simulink model "trajectory_plot"  (R2021a)
settings: Solver=FixedStepAuto  StartTime=0.0  StopTime=sim_time  RelTol=1e-3
values from neighbouring files (symbols this model uses):
  mjd2000_dep = MA.SC1.mjd2000_dep    [main_video_sim.m]
  TrajSC = [TrajSC, time_mjd2000_traj']    [main_video_sim.m]
undefined symbols (not defined in the file or in its folder): adim, planet_eph
libraries: vrlib x1
settings Model: SimulationMode=accelerator  Creator=enric  LastModifiedBy=enric

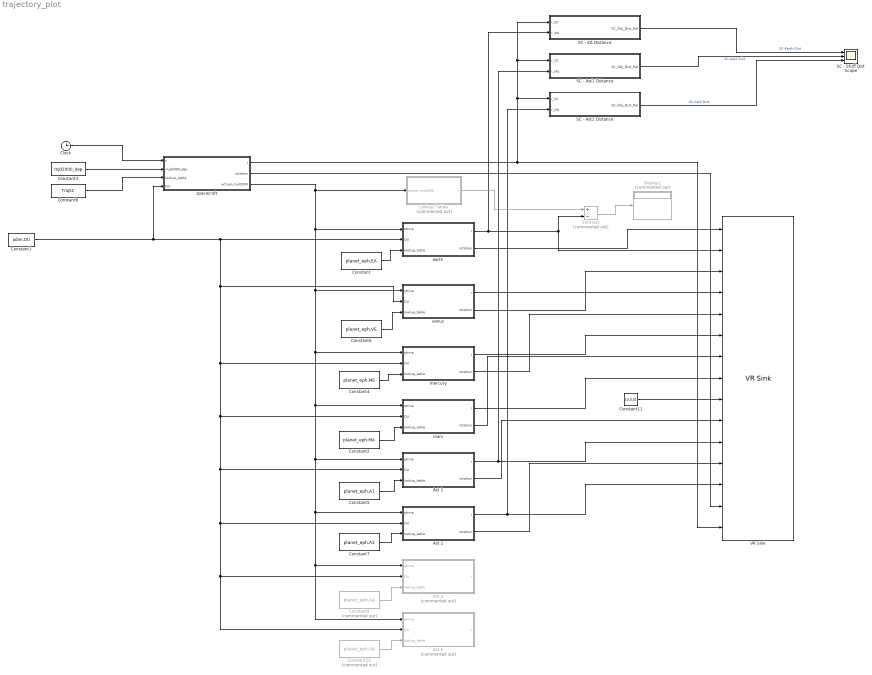
== system trajectory_plot ==
  Ast 1 : MATLAB Function  TreatAsAtomicUnit=on
  Ast 2 : MATLAB Function  TreatAsAtomicUnit=on
  Ast a : MATLAB Function  Commented=on  TreatAsAtomicUnit=on
  Ast b : MATLAB Function  Commented=on  TreatAsAtomicUnit=on
  Clock : Clock
  Constant : Constant  Value=planet_eph.EA
  Constant1 : Constant  Value=adim.DU
  Constant10 : Constant  Commented=on  Value=planet_eph.Ab
  Constant11 : Constant  Value=[0,0,5]
  Constant2 : Constant  Value=planet_eph.MA
  Constant3 : Constant  Value=mjd2000_dep
  Constant4 : Constant  Value=planet_eph.ME
  Constant5 : Constant  Value=planet_eph.A1
  Constant6 : Constant  Value=planet_eph.VE
  Constant7 : Constant  Value=planet_eph.A2
  Constant8 : Constant  Value=TrajSC
  Constant9 : Constant  Commented=on  Value=planet_eph.Aa
  Display1 : Display  Commented=on
  Lookup Tables : Subsystem  Commented=on
  SC - Ast1 Distance : MATLAB Function  TreatAsAtomicUnit=on
  SC - Ast2 Distance : MATLAB Function  TreatAsAtomicUnit=on
  SC - EA Distance : MATLAB Function  TreatAsAtomicUnit=on
  SC - Stuff Dist Scope : Scope  NumInputPorts=3
  Subtract : Sum  Commented=on  Inputs=+-
  VR Sink : vrlib/VR Sink  InstantiateOnLoad=on  SampleTime=0.1  ViewEnable=on  RemoteChange=off  RemoteView=off  FieldsWritten=Earth.rotation.4.1.1.double#Earth.translation.3.1.1.double#Venus.rotation.4.1.1.double#Venus.translation.3.1.1.double#Mercury.rotation.4.1.1.double#Mercury.translation.3.1.1.double#Mars.rotation.4.1.1.double#Mars.translation.3.1.1.double#Luigi.position.3.1.1.double#Golevka.rotation.4.1.1.double#Golevka.translation.3.1.1.double#Tautatis.rotation.4.1.1.double#Tautatis.translation.3.1.1.double#Hayabusa2.rotation.4.1.1.double#Hayabusa2.translation.3.1.1.double  WorldFileName=inner_solar_system.x3d  AutoView=on  VideoDimensions=[]  AllowVariableSize=off
  earth : MATLAB Function  TreatAsAtomicUnit=on
  mars : MATLAB Function  TreatAsAtomicUnit=on
  mercury : MATLAB Function  TreatAsAtomicUnit=on
  spacecraft : MATLAB Function  TreatAsAtomicUnit=on
  venus : MATLAB Function  TreatAsAtomicUnit=on
  wires:
  earth/1(r) -> SC - EA Distance/2(r_obj), VR Sink/2, Subtract/2
  Constant/1 -> earth/3(lookup_table)
  Constant2/1 -> mars/3(lookup_table)
  mars/1(r) -> VR Sink/8
  Constant4/1 -> mercury/3(lookup_table)
  mercury/1(r) -> VR Sink/6
  Constant1/1 -> mars/2(DU), Ast 2/2(DU), Ast b/2(DU), Ast a/2(DU), Ast 1/2(DU), mercury/2(DU), venus/2(DU), earth/2(DU), spacecraft/4(DU)
  Constant6/1 -> venus/3(lookup_table)
  venus/1(r) -> VR Sink/4
  Constant8/1 -> spacecraft/3(lookup_table)
  Clock/1 -> spacecraft/1(t)
  Constant3/1 -> spacecraft/2(mjd2000_dep)
  spacecraft/3(actual_mjd2000) -> earth/1(qtime), mars/1(qtime), Ast 1/1(qtime), Ast 2/1(qtime), Ast b/1(qtime), Ast a/1(qtime), mercury/1(qtime), venus/1(qtime), Lookup Tables/1(actual mjd2000)
  Constant5/1 -> Ast 1/3(lookup_table)
  Constant7/1 -> Ast 2/3(lookup_table)
  Constant9/1 -> Ast a/3(lookup_table)
  Constant10/1 -> Ast b/3(lookup_table)
  Ast 1/1(r) -> VR Sink/11, SC - Ast1 Distance/2(r_obj)
  Ast 2/1(r) -> SC - Ast2 Distance/2(r_obj), VR Sink/13
  spacecraft/1(r) -> VR Sink/15, SC - EA Distance/1(r_SC), SC - Ast1 Distance/1(r_SC), SC - Ast2 Distance/1(r_SC)
  Lookup Tables/1(r) -> Subtract/1
  Subtract/1 -> Display1/1
  earth/2(rotation) -> VR Sink/1
  venus/2(rotation) -> VR Sink/3
  mercury/2(rotation) -> VR Sink/5
  Ast 2/2(rotation) -> VR Sink/12
  Ast 1/2(rotation) -> VR Sink/10
  mars/2(rotation) -> VR Sink/7
  Constant11/1 -> VR Sink/9
  spacecraft/2(rotation) -> VR Sink/14
  SC - EA Distance/1(SC_Obj_Dist_Rel) -> SC - Stuff Dist Scope/1  "SC-Earth Dist"
  SC - Ast1 Distance/1(SC_Obj_Dist_Rel) -> SC - Stuff Dist Scope/2  "SC-Ast1 Dist"
  SC - Ast2 Distance/1(SC_Obj_Dist_Rel) -> SC - Stuff Dist Scope/3  "SC-Ast2 Dist"

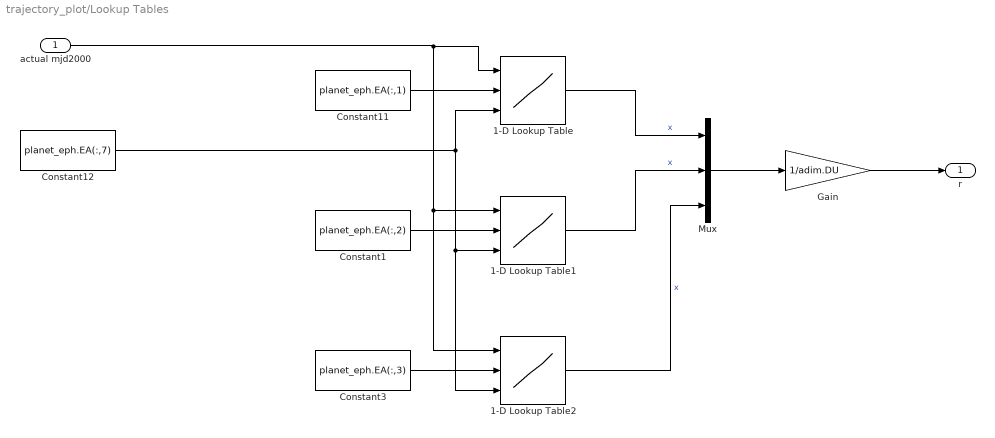
== system trajectory_plot/Lookup Tables ==
  actual mjd2000 : Inport
  1-D Lookup Table : Lookup_n-D  NumberOfTableDimensions=1  BreakpointsForDimension1Source=Input port  BreakpointsForDimension1=[7]  TableSource=Input port  Table=tanh([-5:5])  InternalRulePriority=Speed  RndMeth=Simplest  InputSameDT=on
      settings: InputPortMap=u0,p221,p5
  1-D Lookup Table1 : Lookup_n-D  NumberOfTableDimensions=1  BreakpointsForDimension1Source=Input port  BreakpointsForDimension1=[7]  TableSource=Input port  Table=tanh([-5:5])  InternalRulePriority=Speed  RndMeth=Simplest  InputSameDT=on
      settings: InputPortMap=u0,p221,p5
  1-D Lookup Table2 : Lookup_n-D  NumberOfTableDimensions=1  BreakpointsForDimension1Source=Input port  BreakpointsForDimension1=[7]  TableSource=Input port  Table=tanh([-5:5])  InternalRulePriority=Speed  RndMeth=Simplest  InputSameDT=on
      settings: InputPortMap=u0,p221,p5
  Constant1 : Constant  Value=planet_eph.EA(:,2)
  Constant11 : Constant  Value=planet_eph.EA(:,1)
  Constant12 : Constant  Value=planet_eph.EA(:,7)
  Constant3 : Constant  Value=planet_eph.EA(:,3)
  Gain : Gain  Gain=1/adim.DU
  Mux : Mux  Inputs=3
  r : Outport
  wires:
  actual mjd2000/1 -> 1-D Lookup Table2/1, 1-D Lookup Table1/1, 1-D Lookup Table/1
  Constant11/1 -> 1-D Lookup Table/2
  Gain/1 -> r/1
  Mux/1 -> Gain/1
  1-D Lookup Table/1 -> Mux/1  "x"
  Constant1/1 -> 1-D Lookup Table1/2
  Constant3/1 -> 1-D Lookup Table2/2
  Constant12/1 -> 1-D Lookup Table2/3, 1-D Lookup Table1/3, 1-D Lookup Table/3
  1-D Lookup Table1/1 -> Mux/2  "x"
  1-D Lookup Table2/1 -> Mux/3  "x"

== matlab function trajectory_plot/SC - EA Distance ==
  data: r_SC input; r_obj input; SC_Obj_Dist_Rel output
function SC_Obj_Dist_Rel = SC_Obj_dist(r_SC, r_obj)

SC_Obj_Dist_Rel = sqrt((r_SC(1) - r_obj(1))^2 + (r_SC(2) - r_obj(2))^2 +(r_SC(3) - r_obj(3))^2 );

end

== matlab function trajectory_plot/SC - Ast1 Distance ==
  data: r_SC input; r_obj input; SC_Obj_Dist_Rel output
function SC_Obj_Dist_Rel = SC_Obj_dist(r_SC, r_obj)

SC_Obj_Dist_Rel = sqrt((r_SC(1) - r_obj(1))^2 + (r_SC(2) - r_obj(2))^2 +(r_SC(3) - r_obj(3))^2 );

end

== matlab function trajectory_plot/SC - Ast2 Distance ==
  data: r_SC input; r_obj input; SC_Obj_Dist_Rel output
function SC_Obj_Dist_Rel = SC_Obj_dist(r_SC, r_obj)

SC_Obj_Dist_Rel = sqrt((r_SC(1) - r_obj(1))^2 + (r_SC(2) - r_obj(2))^2 +(r_SC(3) - r_obj(3))^2 );

end

== matlab function trajectory_plot/earth ==
  data: qtime input; DU input; lookup_table input; r output; rotation output
function [r, rotation]  = planet_eph(qtime, DU, lookup_table)

% initialise
r = zeros(3,1);
% v = zeros(3,1);

% assign
r(1:3,1) = interp1(lookup_table(:,7),lookup_table(:,1:3),qtime)/DU;
% v(1:3,1) = interp1(lookup_table(:,7),lookup_table(:,4:6),qtime)/DU*TU;

EarthDay = 23*3600+56*60; % s

w_Earth = 2*pi/EarthDay; % rad/s

tilt_axis = deg2rad(23.4); % rad
rotation = [sin(tilt_axis);sin(tilt_axis);cos(tilt_axis); w_Earth]; % direction 3 componets, magnitude

end

== matlab function trajectory_plot/mars ==
  data: qtime input; DU input; lookup_table input; r output; rotation output
function [r, rotation]  = planet_eph(qtime, DU, lookup_table)

% initialise
r = zeros(3,1);
% v = zeros(3,1);

% assign
r(1:3,1) = interp1(lookup_table(:,7),lookup_table(:,1:3),qtime)/DU;
% v(1:3,1) = interp1(lookup_table(:,7),lookup_table(:,4:6),qtime)/DU*TU;

MarsDay = 24*3600+39*60; % s

w_Mars = 2*pi/MarsDay; % rad/s

tilt_axis = deg2rad(25); % rad
rotation = [sin(tilt_axis);sin(tilt_axis);cos(tilt_axis); w_Mars]; % direction 3 componets, magnitude

end

== matlab function trajectory_plot/mercury ==
  data: qtime input; DU input; lookup_table input; r output; rotation output
function [r, rotation]  = planet_eph(qtime, DU, lookup_table)

% initialise
r = zeros(3,1);
% v = zeros(3,1);

% assign
r(1:3,1) = interp1(lookup_table(:,7),lookup_table(:,1:3),qtime)/DU;
% v(1:3,1) = interp1(lookup_table(:,7),lookup_table(:,4:6),qtime)/DU*TU;

MercuryDay = 58*24*3600+15*3600+30*60+30; % s

w_Mercury = 2*pi/MercuryDay; % rad/s

tilt_axis = 0; % rad
rotation = [sin(tilt_axis);sin(tilt_axis);cos(tilt_axis); w_Mercury]; % direction 3 componets, magnitude

end

== matlab function trajectory_plot/venus ==
  data: qtime input; DU input; lookup_table input; r output; rotation output
function [r, rotation]  = planet_eph(qtime, DU, lookup_table)

% initialise
r = zeros(3,1);
% v = zeros(3,1);

% assign
r(1:3,1) = interp1(lookup_table(:,7),lookup_table(:,1:3),qtime)/DU;
% v(1:3,1) = interp1(lookup_table(:,7),lookup_table(:,4:6),qtime)/DU*TU;

VenusDay = 243*24*3600+26*60; % s

w_Venus = 2*pi/VenusDay; % rad/s

tilt_axis = deg2rad(177); % rad
rotation = [sin(tilt_axis);sin(tilt_axis);cos(tilt_axis); w_Venus]; % direction 3 componets, magnitude

end

== matlab function trajectory_plot/spacecraft ==
  data: t input; mjd2000_dep input; lookup_table input; DU input; r output; rotation output; actual_mjd2000 output
function [r, rotation, actual_mjd2000]  = sc_trajectory(t, mjd2000_dep, lookup_table, DU)

% t [days]
actual_mjd2000 = mjd2000_dep + t;

% initialise
r = zeros(3,1);
% v = zeros(3,1);

% assign
r(1:3,1) = interp1(lookup_table(:,4),lookup_table(:,1:3),actual_mjd2000)/DU;
% v(1:3,1) = interp1(lookup_table(:,7),lookup_table(:,4:6),qtime)/DU*TU;

SC_period = 23*3600+56*60; % s

w_SC = 2*pi/SC_period; % rad/s

tilt_axis = deg2rad(0); % rad
rotation = [sin(tilt_axis);sin(tilt_axis);cos(tilt_axis); w_SC]; % direction 3 componets, magnitude

end

== matlab function trajectory_plot/Ast 1 ==
  data: qtime input; DU input; lookup_table input; r output; rotation output
function [r, rotation]  = planet_eph(qtime, DU, lookup_table)

% initialise
r = zeros(3,1);
% v = zeros(3,1);

% assign
r(1:3,1) = interp1(lookup_table(:,7),lookup_table(:,1:3),qtime)/DU;
% v(1:3,1) = interp1(lookup_table(:,7),lookup_table(:,4:6),qtime)/DU*TU;

Ast1Day = 24*3600; % s --------- set

w_Ast1 = 2*pi/Ast1Day; % rad/s

tilt_axis = deg2rad(0); % rad ---------- set
rotation = [sin(tilt_axis);sin(tilt_axis);cos(tilt_axis); w_Ast1]; % direction 3 componets, magnitude

end

== matlab function trajectory_plot/Ast 2 ==
  data: qtime input; DU input; lookup_table input; r output; rotation output
function [r, rotation]  = planet_eph(qtime, DU, lookup_table)

% initialise
r = zeros(3,1);
% v = zeros(3,1);

% assign
r(1:3,1) = interp1(lookup_table(:,7),lookup_table(:,1:3),qtime)/DU;
% v(1:3,1) = interp1(lookup_table(:,7),lookup_table(:,4:6),qtime)/DU*TU;

Ast2Day = 24*3600; % s --------- set

w_Ast2 = 2*pi/Ast2Day; % rad/s

tilt_axis = deg2rad(0); % rad ---------- set
rotation = [sin(tilt_axis);sin(tilt_axis);cos(tilt_axis); w_Ast2]; % direction 3 componets, magnitude

end

== matlab function trajectory_plot/Ast a ==
  data: qtime input; DU input; lookup_table input; r output
function r  = planet_eph(qtime, DU, lookup_table)

% initialise
r = zeros(3,1);
% v = zeros(3,1);

% assign
r(1:3,1) = interp1(lookup_table(:,7),lookup_table(:,1:3),qtime)/DU;
% v(1:3,1) = interp1(lookup_table(:,7),lookup_table(:,4:6),qtime)/DU*TU;

end

== matlab function trajectory_plot/Ast b ==
  data: qtime input; DU input; lookup_table input; r output
function r  = planet_eph(qtime, DU, lookup_table)

% initialise
r = zeros(3,1);
% v = zeros(3,1);

% assign
r(1:3,1) = interp1(lookup_table(:,7),lookup_table(:,1:3),qtime)/DU;
% v(1:3,1) = interp1(lookup_table(:,7),lookup_table(:,4:6),qtime)/DU*TU;

end
